simulink model "new_framework"  (R2020b)
settings: Solver=FixedStepAuto  StartTime=0.0  StopTime=20.0  FixedStep=1e-2  RelTol=1e-3
libraries: simulink x1
settings Model: Creator=Admin  LastModifiedBy=Admin

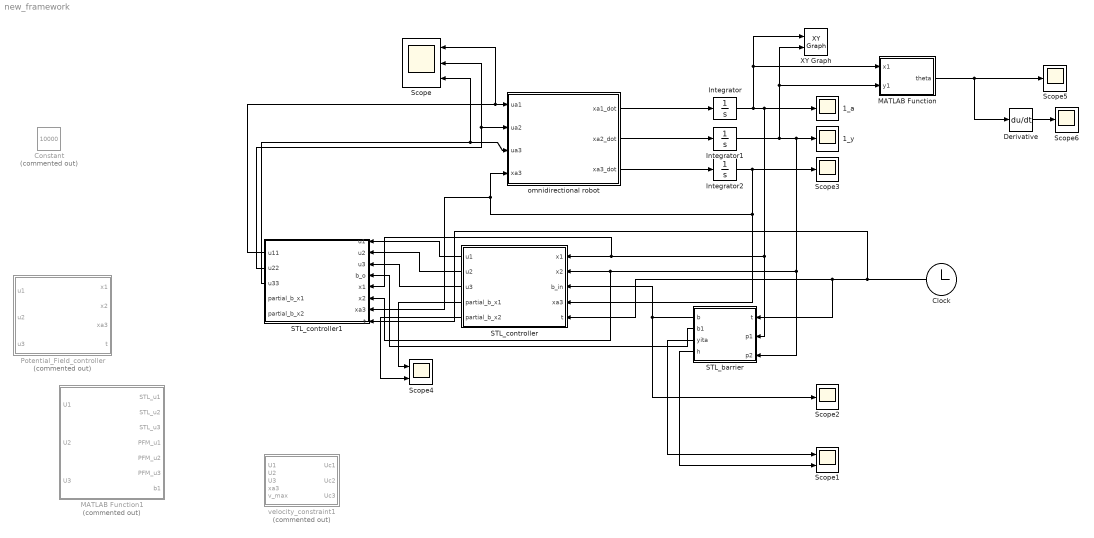
== system new_framework ==
  1_a : Scope
  1_y : Scope
  Clock : Clock
  Constant : Constant  Commented=on  Value=10000
  Derivative : Derivative
  Integrator : Integrator
  Integrator1 : Integrator
  Integrator2 : Integrator
  MATLAB Function : MATLAB Function  TreatAsAtomicUnit=on
  MATLAB Function1 : MATLAB Function  Commented=on  TreatAsAtomicUnit=on
  Potential_Field_controller : MATLAB Function  Commented=on  TreatAsAtomicUnit=on
  "STL_barrier " : MATLAB Function  TreatAsAtomicUnit=on
  STL_controller : MATLAB Function  TreatAsAtomicUnit=on
  STL_controller1 : MATLAB Function  TreatAsAtomicUnit=on
  Scope : Scope  NumInputPorts=3
  Scope1 : Scope  NumInputPorts=2
  Scope{2..3,5..6} (4 alike) : Scope
  Scope4 : Scope  NumInputPorts=2
  XY Graph : simulink/Sinks/XY Graph  xmin=-15  xmax=100  ymin=-15  ymax=100  st=0.01
  omnidirectional robot : MATLAB Function  TreatAsAtomicUnit=on
  velocity_constraint1 : MATLAB Function  Commented=on  TreatAsAtomicUnit=on
  wires:
  "STL_barrier "/1(b) -> Scope2/1, STL_controller/3(b_in)
  omnidirectional robot/1(xa1_dot) -> Integrator/1
  Derivative/1 -> Scope6/1
  MATLAB Function/1(theta) -> Derivative/1, Scope5/1
  Integrator1/1 -> MATLAB Function/2(y1), XY Graph/2, "STL_barrier "/3(p2), STL_controller1/6(x2), STL_controller/2(x2), 1_y/1
  "STL_barrier "/3(yita) -> Scope1/1
  "STL_barrier "/4(h) -> Scope1/2
  Integrator2/1 -> STL_controller1/7(xa3), omnidirectional robot/4(xa3), STL_controller/4(xa3), Scope3/1
  omnidirectional robot/3(xa3_dot) -> Integrator2/1
  Integrator/1 -> MATLAB Function/1(x1), XY Graph/1, "STL_barrier "/2(p1), STL_controller1/5(x1), STL_controller/1(x1), 1_a/1
  Clock/1 -> STL_controller1/8(t), "STL_barrier "/1(t), STL_controller/5(t)
  omnidirectional robot/2(xa2_dot) -> Integrator1/1
  STL_controller/4(partial_b_x1) -> Scope4/1
  STL_controller/5(partial_b_x2) -> Scope4/2
  STL_controller1/1(u11) -> Scope/1, omnidirectional robot/1(ua1)
  STL_controller1/2(u22) -> Scope/2, omnidirectional robot/2(ua2)
  STL_controller1/3(u33) -> omnidirectional robot/3(ua3), Scope/3
  STL_controller/1(u1) -> STL_controller1/1(u1)
  STL_controller/2(u2) -> STL_controller1/2(u2)
  STL_controller/3(u3) -> STL_controller1/3(u3)
  "STL_barrier "/2(b1) -> STL_controller1/4(b_o)

== matlab function new_framework/velocity_constraint1 ==
  data: U1 input; Uc1 output; U2 input; U3 input; xa3 input; v_max input; Uc2 output; Uc3 output
function [Uc1,Uc2,Uc3] = fcn(U1,U2,U3,xa3,v_max)

Li=0.2;
Bi=[0,cos(pi/6),-cos(pi/6);
    -1,sin(pi/6),sin(pi/6);
    Li,Li,Li;];

R1=[cos(xa3),-sin(xa3),0;
    sin(xa3),cos(xa3),0;
    0,0,1;];
R=0.02;
gx=R1*inv(Bi')*R;

U=[U1;U2;U3];
V=[0;0;0];
V=gx*U;
if V(1,1)^2+V(2,1)^2<=v_max^2
     U(1,1)= U(1,1);
     U(2,1)= U(2,1);
else 
    U(1,1)=sqrt(v_max^2/(V(1,1)^2+V(2,1)^2))*U(1,1);
    U(2,1)=sqrt(v_max^2/(V(1,1)^2+V(2,1)^2))*U(2,1);
    U(3,1)=sqrt(v_max^2/(V(1,1)^2+V(2,1)^2))*U(3,1);
end

Uc1=U(1,1);
Uc2=U(2,1);
Uc3=U(3,1);

== matlab function new_framework/STL_barrier  ==
  data: b output; b1 output; yita output; h output; t input; p1 input; p2 input
function [b,b1,yita,h] = fcn(t,p1,p2)
d1=90;
d2=90;

d11=30;
d22=0;

obs1=50;
obs2=50;
if t<=20
    b11=125*exp(-0.2295*t)+5-sqrt( (p1-d1)^2 + (p2-d2)^2 );
    b12=sqrt( (p1-obs1)^2 + (p2-obs2)^2 )-15;
%     b=-(1/20)*log(exp(-20*b11)+exp(-20*b12));
    b=b11;
    b1=sqrt( (p1-obs1)^2 + (p2-obs2)^2 )-15;
    yita=-125*exp(-0.2295*t)+5;
    h=10-sqrt( (p1-d1)^2 + (p2-d2)^2 );
else
    b=105*exp(-0.327*(t-15))+5-sqrt( (p1-d11)^2 + (p2-d22)^2 );
    yita=-105*exp(-0.327*(t-15))+5;
    h=10-sqrt( (p1-d11)^2 + (p2-d22)^2 );
    b1=0
end

== matlab function new_framework/omnidirectional robot ==
  data: ua1 input; xa1_dot output; ua2 input; ua3 input; xa3 input; xa2_dot output; xa3_dot output
function [xa1_dot,xa2_dot,xa3_dot]= fcn(ua1,ua2,ua3,xa3)

Li=0.2;
Bi=[0,cos(pi/6),-cos(pi/6);
    -1,sin(pi/6),sin(pi/6);
    Li,Li,Li;];

R1=[cos(xa3),-sin(xa3),0;
    sin(xa3),cos(xa3),0;
    0,0,1;];
R=0.2;

A=R1*inv(Bi')*R*[ua1;ua2;ua3];
xa1_dot=A(1,1);
xa2_dot=A(2,1);
xa3_dot=A(3,1);

== matlab function new_framework/STL_controller ==
  data: x1 input; x2 input; b_in input; u1 output; xa3 input; u2 output; u3 output; t input; partial_b_x1 output; partial_b_x2 output
function [u1,u2,u3,partial_b_x1,partial_b_x2]= fcn(x1, x2, b_in, xa3,t)
coder.extrinsic('quadoptimizer');
%coder.extrinsic('save');
d1=90.0; d2=90.0;
do1=50; do2=50;
d11=30;d22=0;
    b11=125*exp(-0.2295*t)+5-sqrt( (x1-d1)^2 + (x2-d2)^2 );
    b12=sqrt( (x1-do1)^2 + (x2-do2)^2 )-20;
    yita=20;
    b=-(1/yita)*log(exp(-yita*b11)+exp(-yita*b12));
if t<=20
    partial_b=(1/2)*((x1-d1)^2+(x2-d2)^2)^(-1/2);
    partial_b1_x=[-2*partial_b*(x1-d1),-2*partial_b*(x2-d2),0];
    partial_b_x1=0;
    partial_b_x2=0;
else
    partial_b1_x=[0,0,0];
    partial_b_x1=0;
    partial_b_x2=0;
    partial_b_b1=1;
    partial_b=(1/2)*((x1-d11)^2+(x2-d22)^2)^(-1/2);
    partial_b_x=[-2*partial_b*(x1-d11),-2*partial_b*(x2-d22),0];    
end
Li=0.2;
Bi=[0,cos(pi/6),-cos(pi/6);
    -1,sin(pi/6),sin(pi/6);
    Li,Li,Li;];

R1=[cos(xa3),-sin(xa3),0;
    sin(xa3),cos(xa3),0;
    0,0,1;];
R=0.2;

gx=R1*inv(Bi')*R;

A=partial_b1_x*gx;

H=[1,0,0;0,1,0;0,0,1];
F=[];
%H=[1];
if t<=20
     b=0.2*b_in-0.2295*125*exp(-0.2295*t);
%     if b_in>0
%     b=1*b_in^2-partial_b_b1*0.2295*125*exp(-0.2295*t)-1;
%     else
%      b=-1*b_in^2-partial_b_b1*0.2295*125*exp(-0.2295*t)-1;
%     end
else
    b=1*b_in-0.327*105*exp(-0.327*(t-15))-1;
end


u1=0;u2=0;u3=0;
U=quadoptimizer(H,b,A,F);

%U=quadprod(H,[],-A,b);

u1=U(1,1);
u2=U(2,1);
u3=U(3,1);

== matlab function new_framework/MATLAB Function ==
  data: x1 input; theta output; y1 input
function theta = fcn(x1, y1)
theta=atan2(y1,x1);

== matlab function new_framework/Potential_Field_controller ==
  data: x1 input; x2 input; u1 output; xa3 input; u2 output; u3 output; t input
function [u1,u2,u3] = fcn(x1, x2, xa3,t)
coder.extrinsic('Calculate_gradient');
coder.extrinsic('PVF_optimizer');
coder.extrinsic('add_random');
A1=[-1,0;0,-1];
if t<15
    F=[180,180];
else
    F=[60,0];
end
distance=sqrt((x1-90)^2+(x2-90)^2);
gradient_x=0;gradient_y=0;
[gradient_x,gradient_y]=Calculate_gradient(x1,x2,A1,F,50,50,20);
% gradient_x=Gradient(1,1);
% gradient_y=Gradient(1,2);
gradient_z=0;
Gradient_all=[gradient_x;gradient_y;gradient_z];

Li=0.2;
Bi=[0,cos(pi/6),-cos(pi/6);
    -1,sin(pi/6),sin(pi/6);
    Li,Li,Li;];

R1=[cos(xa3),-sin(xa3),0;
    sin(xa3),cos(xa3),0;
    0,0,1;];
R=0.02;
gx=R1*inv(Bi')*R;
A=Gradient_all'*gx;

%H=[1];
%H=[1,0;0,1];
%H=[0,0,0;0,0,0;0,0,0];
% H=[1,0,0;0,1,0;0,0,1];
 H=(1/2)*gx'*gx;
b=[0];
F=[-2*gx'*50*Gradient_all];
%=[];
u1=0;u2=0;u3=0;
U=PVF_optimizer(H,b,A,F,distance,gradient_x,gradient_y);

u1=U(1,1);
u2=U(2,1);
u3=U(3,1);

== matlab function new_framework/MATLAB Function1 ==
  data: STL_u1 input; U1 output; STL_u2 input; STL_u3 input; PFM_u1 input; PFM_u2 input; PFM_u3 input; b1 input; U2 output; U3 output
function [U1,U2,U3] = fcn(STL_u1,STL_u2,STL_u3,PFM_u1,PFM_u2,PFM_u3,b1)
U_goal=[STL_u1;STL_u2;STL_u3];
U_obs=[PFM_u1;PFM_u2;PFM_u3];
k=0.15;
lambda=1-exp(-k*max(b1,0));
% U=lambda*U_goal+(1-lambda)*U_obs;
U=U_goal;
U1=0;U2=0;U3=0;
U1=U(1,1);
U2=U(2,1);
U3=U(3,1);

== matlab function new_framework/STL_controller1 ==
  data: u1 input; u2 input; u3 input; b_o input; x1 input; x2 input; u11 output; xa3 input; u22 output; u33 output; t input; partial_b_x1 output; partial_b_x2 output
function [u11,u22,u33,partial_b_x1,partial_b_x2]= fcn(u1, u2, u3, b_o,x1,x2, xa3,t)
coder.extrinsic('quadoptimizer');
%coder.extrinsic('save');
d1=90.0000; d2=90.0000;
do1=50; do2=50;
d11=30;d22=0;
    b11=125*exp(-0.2295*t)+5-sqrt( (x1-d1)^2 + (x2-d2)^2 );
    b12=sqrt( (x1-do1)^2 + (x2-do2)^2 )-15;
    yita=20;
    b=-(1/yita)*log(exp(-yita*b11)+exp(-yita*b12));
if t<=20
    partial_b=(1/2)*((x1-do1)^2+(x2-do2)^2)^(-1/2);
    partial_b1_x=[2*partial_b*(x1-do1),2*partial_b*(x2-do2),0];
    partial_b_x1=0;
    partial_b_x2=0;
else
    partial_b1_x=[0,0,0];
    partial_b2_x=[0,0,0];
    partial_b_x1=0;
    partial_b_x2=0;
    partial_b_b1=1;
    partial_b=(1/2)*((x1-d11)^2+(x2-d22)^2)^(-1/2);
    partial_b_x=[-2*partial_b*(x1-d11),-2*partial_b*(x2-d22),0];    
end
Li=0.2;
Bi=[0,cos(pi/6),-cos(pi/6);
    -1,sin(pi/6),sin(pi/6);
    Li,Li,Li;];

R1=[cos(xa3),-sin(xa3),0;
    sin(xa3),cos(xa3),0;
    0,0,1;];
R=0.2;

gx=R1*inv(Bi')*R;

A=partial_b1_x*gx;

H=[1,0,0;0,1,0;0,0,1];
F=[-2*u1;-2*u2;-2*u3];
%H=[1];
if t<=20
     b=1*b_o;
%     if b_in>0
%     b=1*b_in^2-partial_b_b1*0.2295*125*exp(-0.2295*t)-1;
%     else
%      b=-1*b_in^2-partial_b_b1*0.2295*125*exp(-0.2295*t)-1;
%     end
else
    b=1*b_o-1;
end


u11=0;u22=0;u33=0;
U=quadoptimizer(H,b,A,F);

%U=quadprod(H,[],-A,b);

u11=U(1,1);
u22=U(2,1);
u33=U(3,1);
